simulink model "simulink_3"  (R2016a)
settings: Solver=ode5  StartTime=0.0  StopTime=15.0  FixedStep=0.01  RelTol=1e-3
settings Model: Creator=Abhay  LastModifiedBy=Abhay
settings DataIOCC: LimitDataPoints=on  SaveFormat=Array
settings DebuggingCC: SolverPrmCheckMsg=warning
settings HardwareCC: ProdBitPerPointer=32  ProdLargestAtomicFloat=None  ProdIntDivRoundTo=Undefined  ProdEndianess=Unspecified  ProdWordSize=32  ProdHWDeviceType=32-bit Generic
settings ModelReferenceCC: PropagateSignalLabelsOutOfModel=off
settings ConfigComp: CovModelRefEnable=Off  CovSFcnEnable=off

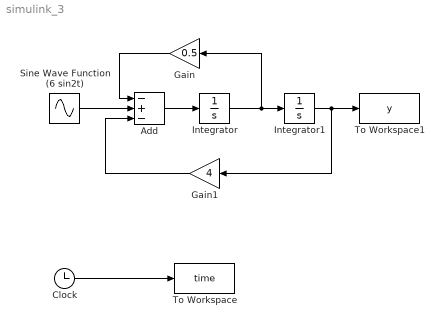
== system simulink_3 ==
  Add : Sum  Inputs=-+-
  Clock : Clock
  Gain : Gain  Gain=0.5
  Gain1 : Gain  Gain=4
  Integrator : Integrator
  Integrator1 : Integrator
  Sine Wave Function (6 sin2t) : Sin  Amplitude=6  Frequency=2  SampleTime=0
  To Workspace : ToWorkspace  VariableName=time  SampleTime=-1
  To Workspace1 : ToWorkspace  VariableName=y  SampleTime=-1
  wires:
  Gain/1 -> Add/1
  Gain1/1 -> Add/3
  Sine Wave Function (6 sin2t)/1 -> Add/2
  Add/1 -> Integrator/1
  Integrator/1 -> Gain/1, Integrator1/1
  Integrator1/1 -> Gain1/1, To Workspace1/1
  Clock/1 -> To Workspace/1
